simulink model "L12_OverflowEffects_FilterExport_R2013b"  (R2013b)
settings: Solver=ode45  SolverMode=SingleTasking  StartTime=0.0  StopTime=10.0  RelTol=1e-3
settings Model: CovMetricSettings=dwe  CovHtmlReporting=off  covSaveCumulativeToWorkspaceVar=off  CovSaveSingleToWorkspaceVar=off  CovExternalEMLEnable=on  Creator=ncleju  LastModifiedBy=ncleju
settings DataIOCC: LimitDataPoints=off  SaveFormat=StructureWithTime  ReturnWorkspaceOutputs=on
settings DebuggingCC: UnderspecifiedInitializationDetection=Simplified  MergeDetectMultiDrivingBlocksExec=error  SolverPrmCheckMsg=none  FrameProcessingCompatibilityMsg=error  SFUnexpectedBacktrackingDiag=error  SFNoUnconditionalDefaultTransitionDiag=error
settings HardwareCC: ProdBitPerPointer=64  ProdLargestAtomicFloat=Float  ProdIntDivRoundTo=Zero  ProdEndianess=LittleEndian  ProdHWDeviceType=Specified
settings ModelReferenceCC: PropagateSignalLabelsOutOfModel=on
settings SFSimCC: SimUseLocalCustomCode=on
settings RTWCC: RTWUseLocalCustomCode=on
settings GRTTargetCC: CodeReplacementLibrary=C99 (ISO)

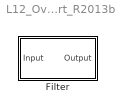
== system L12_OverflowEffects_FilterExport_R2013b ==
  Filter : Subsystem  Tag=FilterWizardSubSystem
      settings: ErrorFcn=dspFilterRealizedInBasicElemsAlgLoopErrFcnCallback

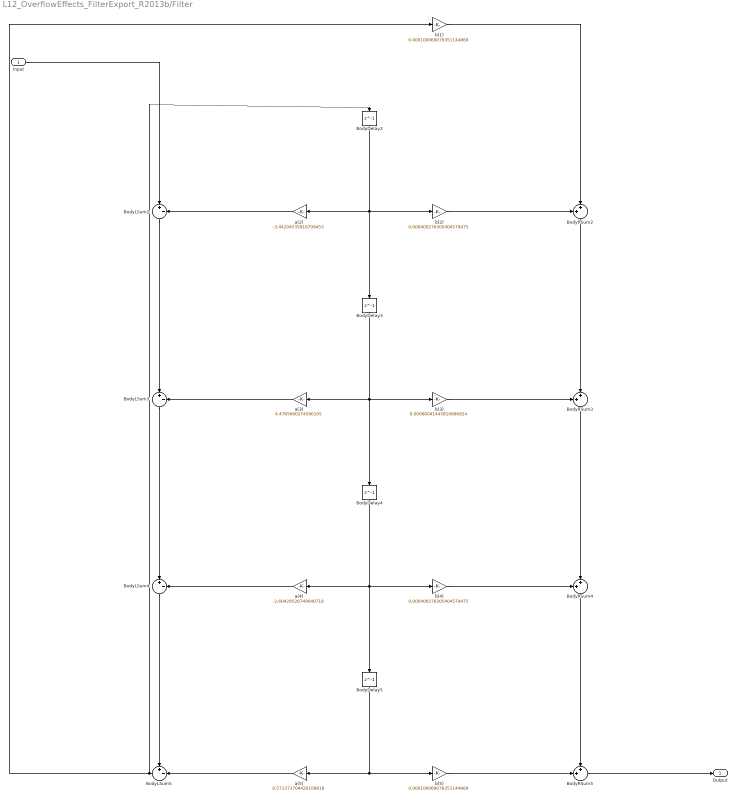
== system L12_OverflowEffects_FilterExport_R2013b/Filter ==
  Input : Inport
  BodyDelay{2..5} (4 alike) : Delay  DelayLength=1  InitialCondition=0
  BodyLSum2 : Sum  Inputs=|+-  RndMeth=Nearest  SaturateOnIntegerOverflow=on  OutDataTypeStr=Inherit: Same as first input
  BodyLSum3 : Sum  Inputs=|+-  RndMeth=Nearest  SaturateOnIntegerOverflow=on  OutDataTypeStr=Inherit: Same as first input
  BodyLSum4 : Sum  Inputs=|+-  RndMeth=Nearest  SaturateOnIntegerOverflow=on  OutDataTypeStr=Inherit: Same as first input
  BodyLSum5 : Sum  Inputs=+-|  RndMeth=Nearest  SaturateOnIntegerOverflow=on  OutDataTypeStr=Inherit: Same as first input
  BodyRSum{2..5} (4 alike) : Sum  Inputs=++|  RndMeth=Nearest  SaturateOnIntegerOverflow=on  OutDataTypeStr=Inherit: Same as first input
  a(2) : Gain  Gain=-3.44204535916709453  ParamDataTypeStr=double  RndMeth=Nearest  SaturateOnIntegerOverflow=on  OutDataTypeStr=Inherit: Same as input
  a(3) : Gain  Gain=4.4765680274590105  ParamDataTypeStr=double  RndMeth=Nearest  SaturateOnIntegerOverflow=on  OutDataTypeStr=Inherit: Same as input
  a(4) : Gain  Gain=-2.60429526749040718  ParamDataTypeStr=double  RndMeth=Nearest  SaturateOnIntegerOverflow=on  OutDataTypeStr=Inherit: Same as input
  a(5) : Gain  Gain=0.571373704420109818  ParamDataTypeStr=double  RndMeth=Nearest  SaturateOnIntegerOverflow=on  OutDataTypeStr=Inherit: Same as input
  b(1) : Gain  Gain=0.000100069076351144869  ParamDataTypeStr=double  RndMeth=Nearest  SaturateOnIntegerOverflow=on  OutDataTypeStr=Inherit: Same as input
  b(2) : Gain  Gain=0.000400276305404579475  ParamDataTypeStr=double  RndMeth=Nearest  SaturateOnIntegerOverflow=on  OutDataTypeStr=Inherit: Same as input
  b(3) : Gain  Gain=0.00060041445810686924  ParamDataTypeStr=double  RndMeth=Nearest  SaturateOnIntegerOverflow=on  OutDataTypeStr=Inherit: Same as input
  b(4) : Gain  Gain=0.000400276305404579475  ParamDataTypeStr=double  RndMeth=Nearest  SaturateOnIntegerOverflow=on  OutDataTypeStr=Inherit: Same as input
  b(5) : Gain  Gain=0.000100069076351144869  ParamDataTypeStr=double  RndMeth=Nearest  SaturateOnIntegerOverflow=on  OutDataTypeStr=Inherit: Same as input
  Output : Outport
  wires:
  b(1)/1 -> BodyRSum2/2
  Input/1 -> BodyLSum2/1
  BodyLSum2/1 -> BodyLSum3/1
  a(2)/1 -> BodyLSum2/2
  BodyDelay2/1 -> a(2)/1, b(2)/1, BodyDelay3/1
  b(2)/1 -> BodyRSum2/1
  BodyRSum2/1 -> BodyRSum3/2
  BodyLSum3/1 -> BodyLSum4/1
  a(3)/1 -> BodyLSum3/2
  BodyDelay3/1 -> a(3)/1, b(3)/1, BodyDelay4/1
  b(3)/1 -> BodyRSum3/1
  BodyRSum3/1 -> BodyRSum4/2
  BodyLSum4/1 -> BodyLSum5/1
  a(4)/1 -> BodyLSum4/2
  BodyDelay4/1 -> a(4)/1, b(4)/1, BodyDelay5/1
  b(4)/1 -> BodyRSum4/1
  BodyRSum4/1 -> BodyRSum5/1
  BodyLSum5/1 -> b(1)/1, BodyDelay2/1
  a(5)/1 -> BodyLSum5/2
  BodyDelay5/1 -> a(5)/1, b(5)/1
  b(5)/1 -> BodyRSum5/2
  BodyRSum5/1 -> Output/1
